simulink model "Drone_Model"  (R2021b)
settings: Solver=VariableStepAuto  StartTime=0.0  StopTime=10  RelTol=1e-3
values from neighbouring files (symbols this model uses):
  G_1 = [ mot_eff,mot_eff,mot_eff,mot_eff;0,-12.8,0,12.8;2.7,0,-2.7,0;-0.115,0.115,-0.115,0.115]./conv    [Model_Parameters.m]    (also in wls_test.m)
  G_2 = [0,0,0,0;0,0,0,0;0,0,0,0;-0.06,0.06,-0.06,0.06]./conv    [Model_Parameters.m]    (also in wls_test.m)
  H_z_den = [1]    [Model_Parameters.m]
  H_z_num = [1]    [Model_Parameters.m]
  mot_den = [1]    [Model_Parameters.m]
  mot_num = [1]    [Model_Parameters.m]
  pseudo_g12 = pinv(G_1+G_2)    [Model_Parameters.m]    (also in wls_test.m)
  Ts = 1/500    (= 0.002)    [Model_Parameters.m]
libraries: dspsrcs4 x1, simulink x1
settings Model: Creator=Tomaso  LastModifiedBy=tomasodeponti
settings DataIOCC: ExternalInput=H_z_num

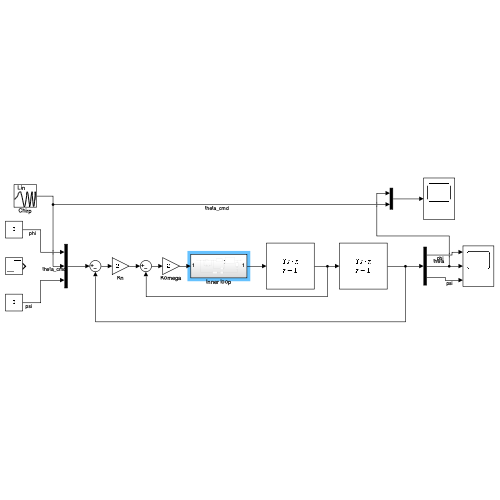
[thumbnail: Simulink's stored preview of the top-level diagram]
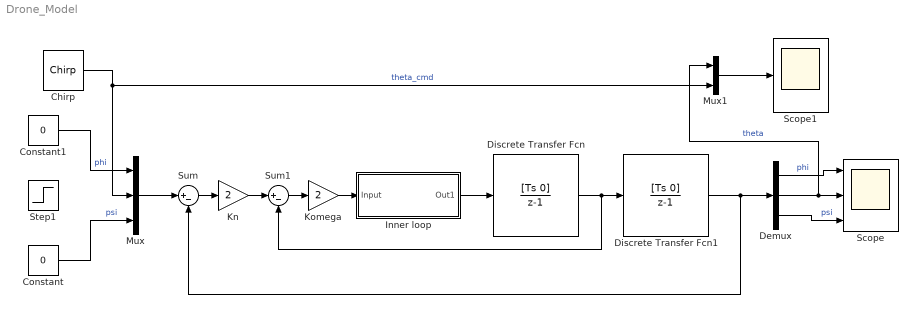
== system Drone_Model ==
  Chirp : dspsrcs4/Chirp  sweep=Linear  mode=Unidirectional  f0=0.1  f1=0.5  t1=0.5  Tsweep=10  phase=0  Ts=1/8000  spf=1  datatype=Double  OutputFrames=off
  Constant : Constant  Value=0
  Constant1 : Constant  Value=0
  Demux : Demux  Outputs=3
  Discrete Transfer Fcn : DiscreteTransferFcn  Numerator=[Ts 0]  Denominator=[1 -1]
  Discrete Transfer Fcn1 : DiscreteTransferFcn  Numerator=[Ts 0]  Denominator=[1 -1]
  Inner loop : Subsystem
  Kn : Gain  Gain=2
  Komega : Gain  Gain=2
  Mux : Mux  Inputs=3
  Mux1 : Mux  Inputs=2
  Scope : Scope  NumInputPorts=3
  Scope1 : Scope
  Step1 : Step  Time=10  SampleTime=0
  Sum : Sum  Inputs=|+-
  Sum1 : Sum  Inputs=|+-
  wires:
  Constant1/1 -> Mux/1  "phi"
  Chirp/1 -> Mux/2, Mux1/2  "theta_cmd"
  Constant/1 -> Mux/3  "psi"
  Inner loop/1(Out1) -> Discrete Transfer Fcn/1
  Discrete Transfer Fcn/1 -> Sum1/2, Discrete Transfer Fcn1/1
  Discrete Transfer Fcn1/1 -> Sum/2, Demux/1
  Demux/1 -> Scope/1  "phi"
  Demux/2 -> Mux1/1, Scope/2  "theta"
  Demux/3 -> Scope/3  "psi"
  Mux/1 -> Sum/1
  Kn/1 -> Sum1/1
  Sum/1 -> Kn/1
  Sum1/1 -> Komega/1
  Komega/1 -> Inner loop/1(Input)
  Mux1/1 -> Scope1/1

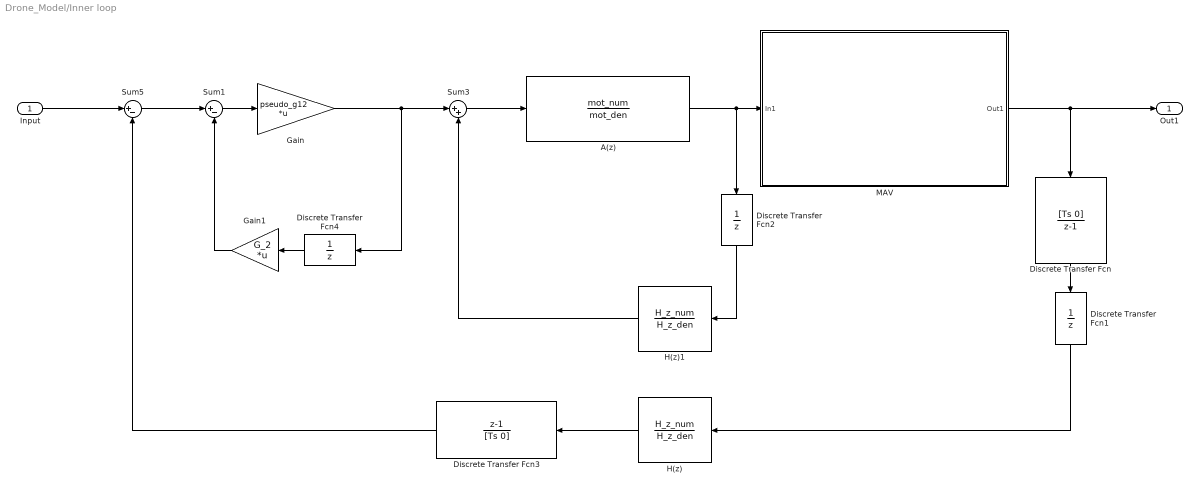
== system Drone_Model/Inner loop ==
  Input : Inport  PortDimensions=3
  A(z) : DiscreteTransferFcn  Numerator=mot_num  Denominator=mot_den  DenCoefDataTypeStr=int16
  Discrete Transfer Fcn : DiscreteTransferFcn  Numerator=[Ts 0]  Denominator=[1 -1]
  Discrete Transfer Fcn1 : DiscreteTransferFcn  Denominator=[1 0]
  Discrete Transfer Fcn2 : DiscreteTransferFcn  Denominator=[1 0]
  Discrete Transfer Fcn3 : DiscreteTransferFcn  Numerator=[1 -1]  Denominator=[Ts 0]
  Discrete Transfer Fcn4 : DiscreteTransferFcn  Denominator=[1 0]
  Gain : Gain  Gain=pseudo_g12  Multiplication=Matrix(K*u)
  Gain1 : Gain  Gain=G_2  Multiplication=Matrix(K*u)
  H(z) : DiscreteTransferFcn  Numerator=H_z_num  Denominator=H_z_den  DenCoefDataTypeStr=int16
  H(z)1 : DiscreteTransferFcn  Numerator=H_z_num  Denominator=H_z_den  DenCoefDataTypeStr=int16
  MAV : Subsystem
      mask Display: image('C:\Users\Tomaso\Pictures\Screenshots\Screenshot 2021-12-02 165056.png'); % Use "Edit Image" on toolstrip to change.
  Sum1 : Sum  Inputs=|+-
  Sum3 : Sum  Inputs=|++
  Sum5 : Sum  Inputs=|+-
  Out1 : Outport  PortDimensions=3
  wires:
  A(z)/1 -> Discrete Transfer Fcn2/1, MAV/1(In1)
  MAV/1(Out1) -> Out1/1, Discrete Transfer Fcn/1
  Discrete Transfer Fcn/1 -> Discrete Transfer Fcn1/1
  Discrete Transfer Fcn1/1 -> H(z)/1
  Discrete Transfer Fcn2/1 -> H(z)1/1
  Sum3/1 -> A(z)/1
  H(z)1/1 -> Sum3/2
  H(z)/1 -> Discrete Transfer Fcn3/1
  Discrete Transfer Fcn3/1 -> Sum5/2
  Gain/1 -> Sum3/1, Discrete Transfer Fcn4/1
  Sum5/1 -> Sum1/1
  Sum1/1 -> Gain/1
  Discrete Transfer Fcn4/1 -> Gain1/1
  Gain1/1 -> Sum1/2
  Input/1 -> Sum5/1

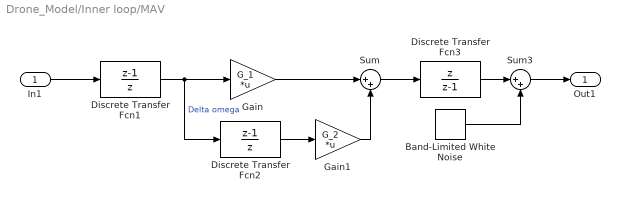
== system Drone_Model/Inner loop/MAV ==
  In1 : Inport  PortDimensions=4
  Band-Limited White Noise : simulink/Sources/Band-Limited White Noise  Cov=[0.1]  Ts=0.1  seed=[23341]
  Discrete Transfer Fcn1 : DiscreteTransferFcn  Numerator=[1 -1]  Denominator=[1 0]
  Discrete Transfer Fcn2 : DiscreteTransferFcn  Numerator=[1 -1]  Denominator=[1 0]
  Discrete Transfer Fcn3 : DiscreteTransferFcn  Numerator=[1 0]  Denominator=[1 -1]
  Gain : Gain  Gain=G_1  Multiplication=Matrix(K*u)
  Gain1 : Gain  Gain=G_2  Multiplication=Matrix(K*u)
  Sum : Sum  Inputs=|++
  Sum3 : Sum  Inputs=|++
  Out1 : Outport  PortDimensions=3
  wires:
  In1/1 -> Discrete Transfer Fcn1/1
  Discrete Transfer Fcn1/1 -> Discrete Transfer Fcn2/1, Gain/1  "Delta omega"
  Discrete Transfer Fcn2/1 -> Gain1/1
  Gain/1 -> Sum/1
  Gain1/1 -> Sum/2
  Sum/1 -> Discrete Transfer Fcn3/1
  Discrete Transfer Fcn3/1 -> Sum3/1
  Band-Limited White Noise/1 -> Sum3/2
  Sum3/1 -> Out1/1
